simulink model "remake"  (R2026a)
settings: Solver=FixedStepAuto  StopTime=50  FixedStep=0.001
values from neighbouring files (symbols this model uses):
  brake_bias_f = 0.60    (= 0.6)    [setupParams.m]    (also in setupParamsSingle.m)
  brake_bias_r = 1 - brake_bias_f    (= 0.4)    [setupParams.m]    (also in setupParamsSingle.m)
  camber_front = -1.5    [setupParams.m]    (also in setupParamsSingle.m)
  camber_rear = -1    [setupParams.m]    (also in setupParamsSingle.m)
  gnd_displ = 0.0    (= 0)    [setupParams.m]    (also in setupParamsSingle.m)
  l_f = 0.775    [setupParams.m]    (also in setupParamsSingle.m)
  l_r = 0.775    [setupParams.m]    (also in setupParamsSingle.m)
  pa_front_wheel = 82700    [setupParams.m]    (also in setupParamsSingle.m)
  pa_rear_wheel = 82700    [setupParams.m]    (also in setupParamsSingle.m)
  scale_factor_front = ones(27, 1)    [setupParams.m]    (also in setupParamsSingle.m)
  scale_factor_rear = ones(27, 1)    [setupParams.m]    (also in setupParamsSingle.m)
  track_width_f = 1.2    [setupParams.m]    (also in setupParamsSingle.m)
  track_width_r = 1.2    [setupParams.m]    (also in setupParamsSingle.m)
  Ts = 0.01    [setupParams.m]    (also in setupParamsSingle.m)
libraries: simulink x30, vehdynlibtire x4, sim3dlib x1, vehdynlibsteering x1, autolibshared x1, sim3dautolib x1
(part 3 of 3)

== matlab function remake/Body/MATLAB Function ==
  data: delta_L input; delta_R input; Fx_FL input; FwF output; Fy_FL input; Fx_FR input; Fy_FR input; Fx_RL input; Fy_RL input; Fx_RR input; Fy_RR input; FwR output
function [FwF, FwR] = rotationary_forces(delta_L, delta_R, Fx_FL, Fy_FL, Fx_FR, Fy_FR, Fx_RL, Fy_RL, Fx_RR, Fy_RR)
    
    % 1. Ruota le forze della ruota Anteriore Sinistra (FL) usando l'angolo sinistro (delta_L)
    Fx_veh_FL = Fx_FL * cos(delta_L) - Fy_FL * sin(delta_L);
    Fy_veh_FL = Fx_FL * sin(delta_L) + Fy_FL * cos(delta_L);

    % 2. Ruota le forze della ruota Anteriore Destra (FR) usando l'angolo destro (delta_R)
    Fx_veh_FR = Fx_FR * cos(delta_R) - Fy_FR * sin(delta_R);
    Fy_veh_FR = Fx_FR * sin(delta_R) + Fy_FR * cos(delta_R);


FwF = [Fx_veh_FL, -Fy_veh_FL;
       Fx_veh_FR, -Fy_veh_FR];

FwR = [Fx_RL, -Fy_RL;
       Fx_RR, -Fy_RR];
end

== matlab function remake/Body/car2wheels ==
  data: delta_L input; delta_R input; Vx input; Vx_hub output; Vy input; yaw_rate input; Vy_hub output; track_width_f parameter; track_width_r parameter; l_f parameter; l_r parameter
function [Vx_hub, Vy_hub] = wheel_kinematics(delta_L, delta_R, Vx, Vy, yaw_rate, track_width_f, track_width_r, l_f, l_r)
% Trasforma le velocità del baricentro (CG) nelle velocità locali dei mozzi ruota.
%
% INPUTS:
% Vx, Vy  : Velocità longitudinali e laterali del veicolo (CG) [m/s]
% yaw_rate       : Velocità di imbardata (yaw_rate ) [rad/s]
% delta_L : Angolo di sterzo ruota anteriore sinistra [rad]
% delta_R : Angolo di sterzo ruota anteriore destra [rad]
% l_f, l_r: Distanza baricentro - asse anteriore/posteriore [m]
% track_width_f, track_width_r: Carreggiata (Track width) anteriore/posteriore [m]
%
% OUTPUTS:
% Vx_hub  : Vettore [FL, FR, RL, RR] delle velocità longitudinali dei mozzi [m/s]
% Vy_hub  : Vettore [FL, FR, RL, RR] delle velocità laterali dei mozzi [m/s]

    %% 1. Velocità nel sistema di riferimento del telaio (non ruotate)
    % Anteriore Sinistra (Front Left)
    V_xf_FL = Vx - (yaw_rate * track_width_f / 2);
    V_yf_FL = Vy + (yaw_rate * l_f);
    
    % Anteriore Destra (Front Right)
    V_xf_FR = Vx + (yaw_rate * track_width_f / 2);
    V_yf_FR = Vy + (yaw_rate * l_f);
    
    % Posteriore Sinistra (Rear Left)
    V_xr_RL = Vx - (yaw_rate * track_width_r / 2);
    V_yr_RL = Vy - (yaw_rate * l_r);
    
    % Posteriore Destra (Rear Right)
    V_xr_RR = Vx + (yaw_rate * track_width_r / 2);
    V_yr_RR = Vy - (yaw_rate * l_r);

    %% 2. Rotazione nel sistema di riferimento della gomma (tramite angolo di sterzo)
    % Le ruote anteriori sono sterzanti
    Vx_FL =  V_xf_FL * cos(delta_L) + V_yf_FL * sin(delta_L);
    Vy_FL = -V_xf_FL * sin(delta_L) + V_yf_FL * cos(delta_L);
    
    Vx_FR =  V_xf_FR * cos(delta_R) + V_yf_FR * sin(delta_R);
    Vy_FR = -V_xf_FR * sin(delta_R) + V_yf_FR * cos(delta_R);
    
    % Le ruote posteriori solitamente non sterzano (delta = 0, quindi cos(0)=1, sin(0)=0)
    Vx_RL = V_xr_RL;
    Vy_RL = V_yr_RL;
    
    Vx_RR = V_xr_RR;
    Vy_RR = V_yr_RR;

    Vx_hub = [Vx_FL; Vx_FR; Vx_RL; Vx_RR];
    Vy_hub = [Vy_FL; Vy_FR; Vy_RL; Vy_RR];
end
